simulink library "ChimePoolDelayLibBtc"  (R2022b)
settings: Solver=VariableStepAuto  StartTime=0.0  StopTime=10.0  RelTol=1e-3
undefined symbols (not defined in the file or in its folder): delay, Row
libraries: TuneVar x2, TOP x1, FeaturePath x1, HandyTextFile x1, RTC x1
settings Model: Creator=kl13806  LastModifiedBy=kl13806
settings SolverCC: AlgebraicLoopSolver=TrustRegion
settings DebuggingCC: UnconnectedInputMsg=warning  UnconnectedOutputMsg=warning  UnconnectedLineMsg=warning  SFMachineParentedDataDiag=warning
settings ModelReferenceCC: EnableRefExpFcnMdlSchedulingChecks=on
settings RTWCC: DLArmComputeVersion=19.05

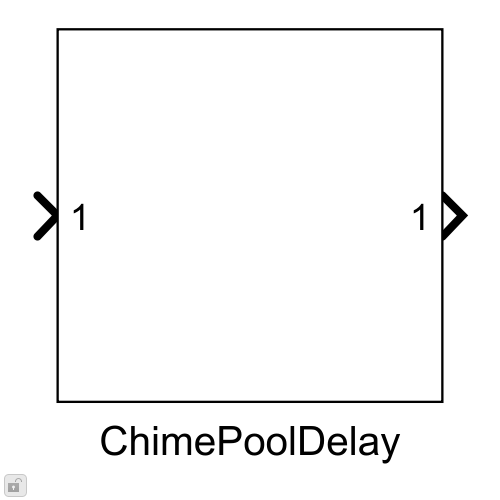
[thumbnail: Simulink's stored preview of the top-level diagram]
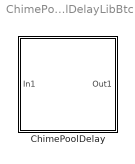
== system ChimePoolDelayLibBtc ==
  ChimePoolDelay : Subsystem  mask(Chimes ChimePoolDelay){Config=[], FeatureName=annDelay}
      mask prompts: Config "ChimePoolDelayConfig"; FeatureName "Feature path name:"
      mask help: Originally part of ChimeExternalProcess, broken into separate library as part of BTC upgrade
      mask init:
      | blkh=gcbh;
      | Config=BTConfig.Assert(blkh,Config);
      | 
      | Config.Validate();
      | BTConfig.InitSetFeatureIfPresent(blkh,'FeatureName');
      mask Callback Config: BTConfig.CallbackHideIfPresent(gcbh,{'FeatureName'});
      mask TypeOptions FeatureName: FeaturePath/FeatureName

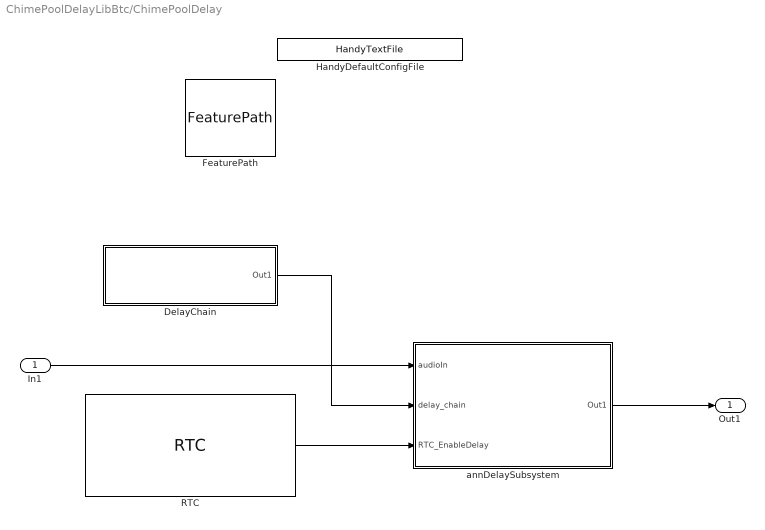
== system ChimePoolDelayLibBtc/ChimePoolDelay ==
  In1 : Inport
  DelayChain : Subsystem
  FeaturePath : FeaturePath/FeaturePath  FeatureName=annDelay  IsGroup=off  GroupNumber=-1  IsModule=off  TriggerInit=[-35 -101 55 -24]
      settings: SourceProductName=Bose Talaria
  HandyDefaultConfigFile : HandyTextFile/HandyTextFile  TemplateSource=Config  FileSuffix=Init  OpenDialogOnLoad=off  UseThisBlockName=off  AddGrandParentNamePrefix=off  TheDefaultText=|  ShowInLibBrowser=on
      | % $(FILENAME) Setup model parameters for each "Init" callback (e.g. update diagram)
      | sample_rate_in_hertz = 44100;
      | frame_size = 32;
      | sysin_channel_count = 2;
      settings: SourceProductName=Bose Talaria
  RTC : RTC/RTC  REQ_Priority=RTC_Mask.NormalPriority  RequestAtInit=off  EnableRequest=off  REQElemName1=Enable_annDelay  REQElemType1=uint32  REQElemWidth1=1  REQElemInitial1=Config.InitialEnableDelay  REQElemType2=uint32  REQElemWidth2=1  REQElemInitial2=[]  REQElemType3=uint32  REQElemWidth3=1  REQElemInitial3=[]  REQElemType4=uint32  REQElemWidth4=1  REQElemInitial4=[]  REQElemType5=uint32  REQElemWidth5=1  REQElemInitial5=[]  REQElemType6=uint32  REQElemWidth6=1  REQElemInitial6=[]  REQElemType7=uint32  REQElemWidth7=1  REQElemInitial7=[]  REQElemType8=uint32  REQElemWidth8=1  REQElemInitial8=[]  REQElemType9=uint32  REQElemWidth9=1  REQElemInitial9=[]  REQElemType10=uint32  REQElemWidth10=1  REQElemInitial10=[]  EnableResponse=on  EnableRSP_StatusIn=off  RSPElemType1=uint32  RSPElemWidth1=1  RSPElemType2=uint32  RSPElemWidth2=1  RSPElemType3=uint32  RSPElemWidth3=1  RSPElemType4=uint32  RSPElemWidth4=1  RSPElemType5=uint32  RSPElemWidth5=1  RSPElemType6=uint32  RSPElemWidth6=1  RSPElemType7=uint32  RSPElemWidth7=1  RSPElemType8=uint32  RSPElemWidth8=1  RSPElemType9=uint32  RSPElemWidth9=1  RSPElemType10=uint32  RSPElemWidth10=1  EnableNotification=off  EnableNTF_PrepTrig=off  NTFElemType1=uint32  NTFElemWidth1=1  NTFElemType2=uint32  NTFElemWidth2=1  NTFElemType3=uint32  NTFElemWidth3=1  NTFElemType4=uint32  NTFElemWidth4=1  NTFElemType5=uint32  NTFElemWidth5=1  NTFElemType6=uint32  NTFElemWidth6=1  NTFElemType7=uint32  NTFElemWidth7=1  NTFElemType8=uint32  NTFElemWidth8=1  NTFElemType9=uint32  NTFElemWidth9=1  NTFElemType10=uint32  NTFElemWidth10=1  MaskMessageName=Enable_Delay
      settings: SourceProductName=Bose Talaria
  annDelaySubsystem : Subsystem
  Out1 : Outport  VectorParamsAs1DForOutWhenUnconnected=off
  wires:
  annDelaySubsystem/1(Out1) -> Out1/1
  RTC/1 -> annDelaySubsystem/3(RTC_EnableDelay)
  DelayChain/1(Out1) -> annDelaySubsystem/2(delay_chain)
  In1/1 -> annDelaySubsystem/1(audioIn)

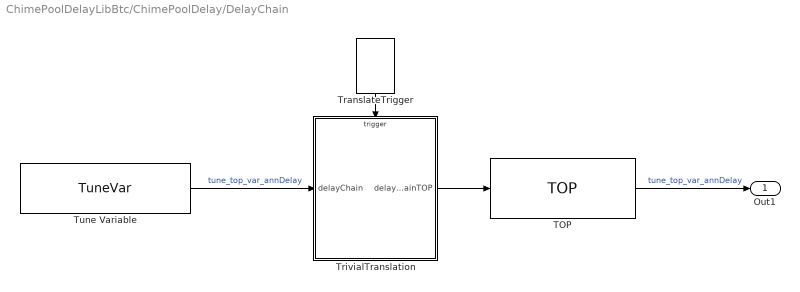
== system ChimePoolDelayLibBtc/ChimePoolDelay/DelayChain ==
  TOP : TOP/TOP  TriggerInit=[440 20 585 80]  TopName=tune_top_var_annDelay  DataType=uint32  BankNumber=0  PreOverlay=false  PostOverlay=false  Role=Automatic
      settings: SourceProductName=Bose Talaria
  TranslateTrigger : TuneVar/TranslateTrigger  TriggerInit=[306 -100 344 -45]
      settings: SourceProductName=Bose Talaria
  TrivialTranslation : MATLAB Function  TreatAsAtomicUnit=on  mask(Talaria Translation){MaxDelay=Config.MaxDelay, NumChannels=Config.NumChannels}
      mask prompts: MaxDelay "Maximum total delay"; NumChannels "Num Channels"
      mask help: This MATLAB Function Block can be automatically inserted by several automation routines. Once placed, the block is ready to accept translation logic from the model designer.
  Tune Variable : TuneVar/TuneVar  TuneName=tune_top_var_annDelay  SpecifyMaxSize=on  VariableDim=1 (Row)  MaxSize=[1 Config.NumChannels]  TunabilityNumber=1  MinValue=[]  MaxValue=[]  TriggerInit=[-30 25 140 75]  MaskValue=Config.DefaultDelayChain
      settings: SourceProductName=Bose Talaria
  Out1 : Outport  VectorParamsAs1DForOutWhenUnconnected=off
  wires:
  TrivialTranslation/1(delayChainTOP) -> TOP/1
  Tune Variable/1 -> TrivialTranslation/1(delayChain)  "tune_top_var_annDelay"
  TOP/1 -> Out1/1  "tune_top_var_annDelay"
  TranslateTrigger/1 -> TrivialTranslation/Trigger

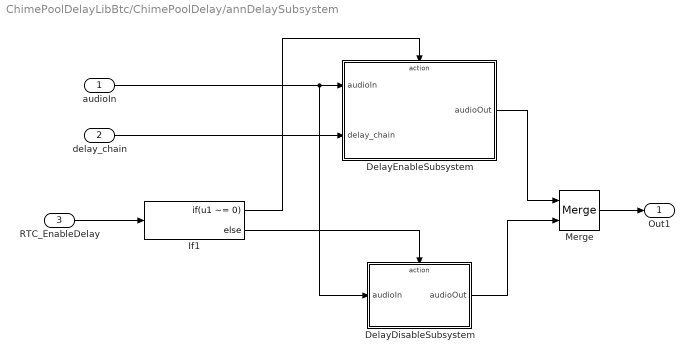
== system ChimePoolDelayLibBtc/ChimePoolDelay/annDelaySubsystem ==
  audioIn : Inport
  delay_chain : Inport  Port=2
  RTC_EnableDelay : Inport  Port=3
  DelayDisableSubsystem : Subsystem  TreatAsAtomicUnit=on
  DelayEnableSubsystem : Subsystem  TreatAsAtomicUnit=on
  If1 : If  IfExpression=u1 ~= 0
  Merge : Merge
  Out1 : Outport  VectorParamsAs1DForOutWhenUnconnected=off
  wires:
  DelayDisableSubsystem/1(audioOut) -> Merge/2
  Merge/1 -> Out1/1
  If1/2 -> DelayDisableSubsystem/Action
  DelayEnableSubsystem/1(audioOut) -> Merge/1
  delay_chain/1 -> DelayEnableSubsystem/2(delay_chain)
  audioIn/1 -> DelayDisableSubsystem/1(audioIn), DelayEnableSubsystem/1(audioIn)
  If1/1 -> DelayEnableSubsystem/Action
  RTC_EnableDelay/1 -> If1/1

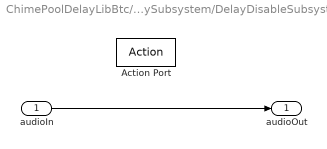
== system ChimePoolDelayLibBtc/ChimePoolDelay/annDelaySubsystem/DelayDisableSubsystem ==
  audioIn : Inport
  Action Port : ActionPort
  audioOut : Outport  VectorParamsAs1DForOutWhenUnconnected=off
  wires:
  audioIn/1 -> audioOut/1

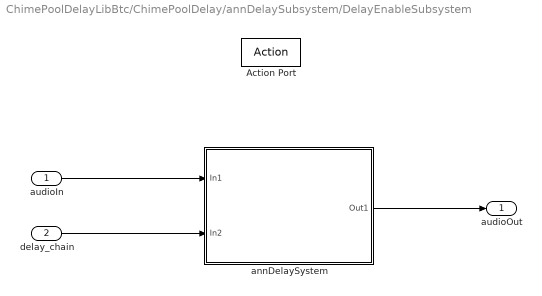
== system ChimePoolDelayLibBtc/ChimePoolDelay/annDelaySubsystem/DelayEnableSubsystem ==
  audioIn : Inport
  delay_chain : Inport  Port=2
  Action Port : ActionPort  ActionPortLabel=if(u1 ~= 0)
  annDelaySystem : Subsystem  TreatAsAtomicUnit=on
  audioOut : Outport  VectorParamsAs1DForOutWhenUnconnected=off
  wires:
  annDelaySystem/1(Out1) -> audioOut/1
  delay_chain/1 -> annDelaySystem/2(In2)
  audioIn/1 -> annDelaySystem/1(In1)

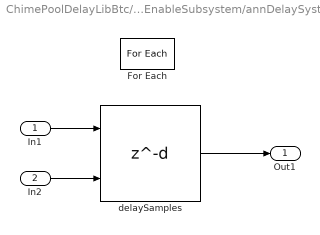
== system ChimePoolDelayLibBtc/ChimePoolDelay/annDelaySubsystem/DelayEnableSubsystem/annDelaySystem ==
  In1 : Inport  Partition=on  PartitionDimension=2  PartitionWidth=1  PartitionOffset=0
  In2 : Inport  Port=2  Partition=on  PartitionDimension=2  PartitionWidth=1  PartitionOffset=0
  For Each : ForEach  DisableCoverage=on
  delaySamples : Delay  DelayLengthSource=Input port  DelayLength=delay  DelayLengthUpperLimit=Config.DefaultMaxDelay  InputProcessing=Columns as channels (frame based)
      settings: InputPortMap=u0,p1
  Out1 : Outport  ConcatenationDimension=2  VectorParamsAs1DForOutWhenUnconnected=off
  wires:
  In1/1 -> delaySamples/1
  delaySamples/1 -> Out1/1
  In2/1 -> delaySamples/2

== matlab function ChimePoolDelayLibBtc/ChimePoolDelay/DelayChain/TrivialTranslation ==
  data: delayChainTOP output; delayChain input; MaxDelay parameter; NumChannels parameter
  events: trigger input FUNCTION_CALL_EVENT
function delayChainTOP  = fcn(delayChain, MaxDelay, NumChannels)
%#codegen

% Verify that the total delay does not exceed the allocated max delay
totalDelay = sum(delayChain.Value);
if (totalDelay > MaxDelay)
    TranslateError('Total delay [%d] must not exceed build-time max [%d]', ...
        totalDelay,MaxDelay);
end

delayChainTOP = delayChain.Value;
